simulink model "Motor0Response"  (R2017a)
settings: Solver=VariableStepAuto  StartTime=0.0  StopTime=1  RelTol=1e-3
undefined symbols (not defined in the file or in its folder): Elec0d, Elec0n, Mech0d, Mech0n, SpdCon0, TCon0
libraries: simulink x1
settings Model: Creator=Matthew  LastModifiedBy=Matthew

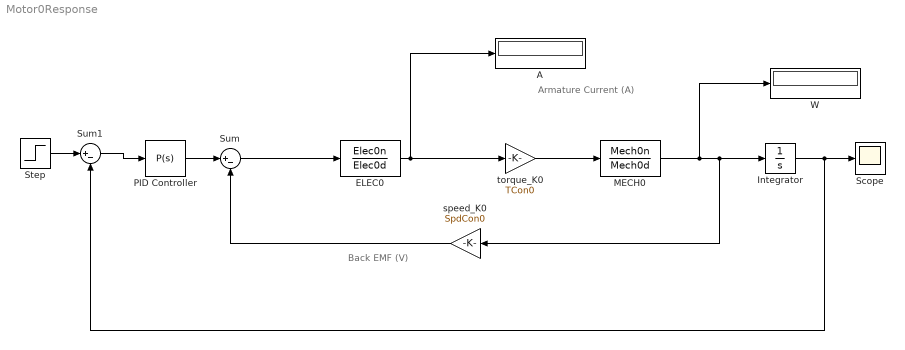
== system Motor0Response ==
  note: Armature Current (A)
  note: Back EMF
      | (V)
  A : Display
  "ELEC0 " : TransferFcn  Numerator=Elec0n  Denominator=Elec0d
  Integrator : Integrator
  "MECH0 " : TransferFcn  Numerator=Mech0n  Denominator=Mech0d
  PID Controller : simulink/Continuous/PID Controller  Controller=P  TimeDomain=Continuous-time  SampleTime=-1  IntegratorMethod=Forward Euler  FilterMethod=Forward Euler  Form=Parallel  UseFilter=on  ControllerParametersSource=internal  P=1.45670718495234  I=1  D=1  N=100  InitialConditionSource=internal  InitialConditionForIntegrator=0  InitialConditionForFilter=0  ExternalReset=none  LimitOutput=off  UpperSaturationLimit=inf  LowerSaturationLimit=-inf  LinearizeAsGain=on  AntiWindupMode=none  Kb=1  TrackingMode=off  Kt=1  PParamMin=[]  PParamMax=[]  IParamMin=[]  IParamMax=[]  DParamMin=[]  DParamMax=[]  NParamMin=[]  NParamMax=[]  KbParamMin=[]  KbParamMax=[]  KtParamMin=[]  KtParamMax=[]  POutMin=[]  POutMax=[]  IOutMin=[]  IOutMax=[]  DOutMin=[]  DOutMax=[]  NOutMin=[]  NOutMax=[]  KbOutMin=[]  KbOutMax=[]  KtOutMin=[]  KtOutMax=[]  IntegratorOutMin=[]  IntegratorOutMax=[]  FilterOutMin=[]  FilterOutMax=[]  SumOutMin=[]  SumOutMax=[]  SumI1OutMin=[]  SumI1OutMax=[]  SumI2OutMin=[]  SumI2OutMax=[]  SumI3OutMin=[]  SumI3OutMax=[]  SumDOutMin=[]  SumDOutMax=[]  SaturationOutMin=[]  SaturationOutMax=[]  IntegratorContinuousStateAttributes=''  IntegratorStateMustResolveToSignalObject=off  IntegratorRTWStateStorageClass=Auto  FilterContinuousStateAttributes=''  FilterStateMustResolveToSignalObject=off  FilterRTWStateStorageClass=Auto  DifferentiatorICPrevScaledInput=0  DifferentiatorOutMin=[]  DifferentiatorOutMax=[]  InitialConditionSetting=State (most efficient)
  Scope : Scope
  Step : Step  Time=0  SampleTime=0
  Sum : Sum  Inputs=|+-
  Sum1 : Sum  Inputs=|+-
  W : Display
  speed_K0 : Gain  Gain=SpdCon0
  torque_K0 : Gain  Gain=TCon0
  wires:
  Step/1 -> Sum1/1
  Sum1/1 -> PID Controller/1
  torque_K0/1 -> "MECH0 "/1
  "ELEC0 "/1 -> torque_K0/1, A/1
  Sum/1 -> "ELEC0 "/1
  speed_K0/1 -> Sum/2
  PID Controller/1 -> Sum/1
  Integrator/1 -> Sum1/2, Scope/1
  "MECH0 "/1 -> W/1, Integrator/1, speed_K0/1
